simulink model "mass_damper"  (R2026a)
settings: Solver=VariableStepAuto
undefined symbols (not defined in the file): c, k, m
settings Model: Creator=mcapoor  LastModifiedBy=mcapoor

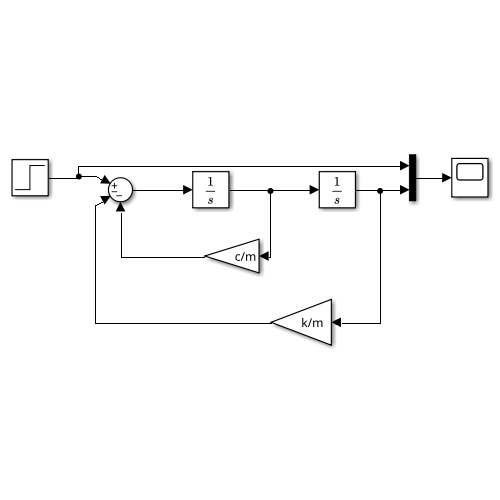
[thumbnail: Simulink's stored preview of the top-level diagram]
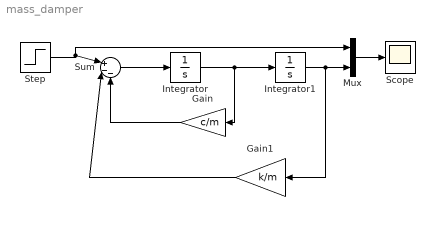
== system mass_damper ==
  Gain : Gain  Gain=c/m
  Gain1 : Gain  Gain=k/m
  Integrator : Integrator
  Integrator1 : Integrator
  Mux : Mux  Inputs=2
  Scope : Scope
      settings: ActiveDisplayYMinimum=-5.6335918062604371  ActiveDisplayYMaximum=4.4037824958156007
  Step : Step  SampleTime=0
  Sum : Sum  Inputs=|+--
  wires:
  Sum/1 -> Integrator/1
  Integrator/1 -> Gain/1, Integrator1/1
  Integrator1/1 -> Mux/2, Gain1/1
  Gain/1 -> Sum/3
  Gain1/1 -> Sum/2
  Step/1 -> Mux/1, Sum/1
  Mux/1 -> Scope/1
